simulink model "examples_of_sine_wave_block"  (R2021a)
settings: Solver=VariableStepAuto  StartTime=0.0  StopTime=1  MaxStep=1e-3  RelTol=1e-3
settings Model: Creator=YasserNet  LastModifiedBy=YasserNet

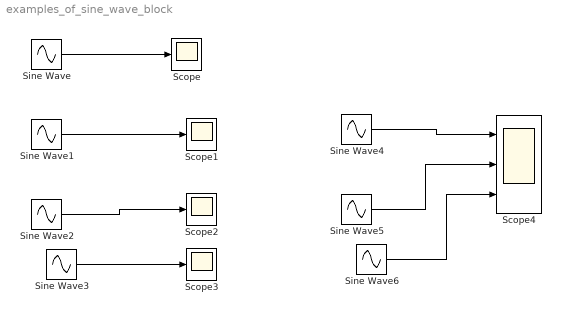
== system examples_of_sine_wave_block ==
  Scope{,1..3} (4 alike) : Scope
  Scope4 : Scope  NumInputPorts=3
  Sine Wave : Sin  Amplitude=5  Frequency=2*pi*2  SampleTime=0
  Sine Wave1 : Sin  Amplitude=10  Frequency=2*pi*5  SampleTime=0
  Sine Wave2 : Sin  Amplitude=10  Frequency=2*pi*5  Phase=-pi  SampleTime=0
  Sine Wave3 : Sin  Amplitude=10  Frequency=2*pi*5  Phase=pi  SampleTime=0
  Sine Wave4 : Sin  Amplitude=10  Frequency=2*pi*5  SampleTime=0
  Sine Wave5 : Sin  Amplitude=10  Frequency=2*pi*5  Phase=-pi  SampleTime=0
  Sine Wave6 : Sin  Amplitude=10  Frequency=2*pi*5  Phase=pi  SampleTime=0
  wires:
  Sine Wave/1 -> Scope/1
  Sine Wave1/1 -> Scope1/1
  Sine Wave2/1 -> Scope2/1
  Sine Wave3/1 -> Scope3/1
  Sine Wave5/1 -> Scope4/2
  Sine Wave6/1 -> Scope4/3
  Sine Wave4/1 -> Scope4/1
